simulink model "ILC_CTC"  (R2023b)
settings: Solver=VariableStepAuto  StartTime=0.0  StopTime=20  RelTol=1e-3
values from neighbouring files (symbols this model uses):
  C1 = [1 0 0 0]    [ILCadaptable.m]    (also in parametros3.m = [1 0 0 0 0 0])
  C2 = [0 1 0 0]    [ILCadaptable.m]    (also in parametros3.m = [0 0 1 0 0 0])
  Cv1 = [0 1 0 0 0 0]    [parametros3.m]
  Cv2 = [0 0 0 1 0 0]    [parametros3.m]
  ek1_1 = out.ek1    [ILCadaptable.m]    (also in parametros3.m)
  ek2_1 = out.ek2    [ILCadaptable.m]    (also in parametros3.m)
  L1 = 2    [ILCadaptable.m]    (also in parametros3.m)
  L2 = 2    [ILCadaptable.m]    (also in parametros3.m)
undefined symbols (not defined in the file or in its folder): l1, l2
libraries: simulink x2
settings Model: Creator=LENOVO  LastModifiedBy=LENOVO

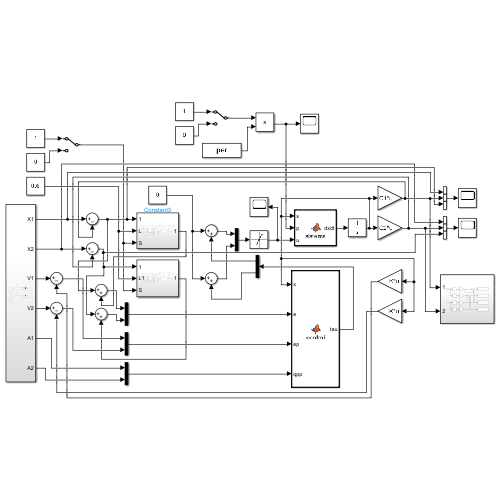
[thumbnail: Simulink's stored preview of the top-level diagram]
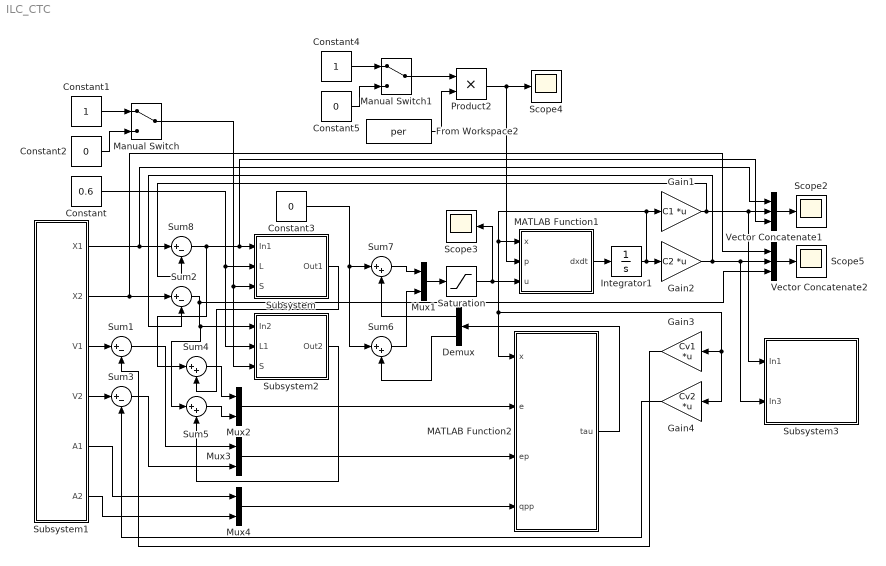
== system ILC_CTC ==
  Constant : Constant  Value=0.6
  Constant1 : Constant
  Constant2 : Constant  Value=0
  Constant3 : Constant  Value=0
  Constant4 : Constant
  Constant5 : Constant  Value=0
  Demux : Demux  Outputs=2
  From Workspace2 : FromWorkspace  VariableName=per
  Gain1 : Gain  Gain=C1  Multiplication=Matrix(K*u)
  Gain2 : Gain  Gain=C2  Multiplication=Matrix(K*u)
  Gain3 : Gain  Gain=Cv1  Multiplication=Matrix(K*u)
  Gain4 : Gain  Gain=Cv2  Multiplication=Matrix(K*u)
  Integrator1 : Integrator  InitialCondition=[0 0 0 0]
  MATLAB Function1 : MATLAB Function  TreatAsAtomicUnit=on
  MATLAB Function2 : MATLAB Function  TreatAsAtomicUnit=on
  Manual Switch : ManualSwitch
  Manual Switch1 : ManualSwitch
  Mux{1..4} (4 alike) : Mux  Inputs=2
  Product2 : Product
  Saturation : Saturate  UpperLimit=2.5  LowerLimit=-2.5
  Scope{2..5} (4 alike) : Scope
  Subsystem : Subsystem
  Subsystem1 : Subsystem
  Subsystem2 : Subsystem
  Subsystem3 : Subsystem
  Sum{1..3,8} (4 alike) : Sum  Inputs=|+-
  Sum{4..7} (4 alike) : Sum  Inputs=|++
  Vector Concatenate1 : Concatenate  NumInputs=3
  Vector Concatenate2 : Concatenate  NumInputs=3
  wires:
  Gain1/1 -> Sum8/2, Subsystem3/1(In1), Vector Concatenate1/2
  Saturation/1 -> Scope3/1, MATLAB Function1/3(u)
  Sum2/1 -> Sum5/1, Subsystem2/1(In2), Vector Concatenate2/3
  Constant1/1 -> Manual Switch/1
  MATLAB Function1/1(dxdt) -> Integrator1/1
  Gain2/1 -> Subsystem3/2(In3), Vector Concatenate2/2, Sum2/2
  Subsystem1/2(X2) -> Sum2/1, Vector Concatenate2/1
  Sum7/1 -> Mux1/1
  Integrator1/1 -> Gain4/1, Gain3/1, MATLAB Function2/1(x), MATLAB Function1/1(x), Gain1/1, Gain2/1
  Vector Concatenate2/1 -> Scope5/1
  Subsystem1/1(X1) -> Vector Concatenate1/1, Sum8/1
  Constant/1 -> Subsystem2/2(L1), Subsystem/2(L)
  Constant2/1 -> Manual Switch/2
  Mux1/1 -> Saturation/1
  Sum8/1 -> Sum4/1, Subsystem/1(In1), Vector Concatenate1/3
  Sum6/1 -> Mux1/2
  Vector Concatenate1/1 -> Scope2/1
  Manual Switch/1 -> Subsystem2/3(S), Subsystem/3(S)
  Subsystem1/3(V1) -> Sum1/1
  Subsystem1/4(V2) -> Sum3/1
  Sum1/1 -> Mux3/1
  Sum3/1 -> Mux3/2
  Subsystem1/5(A1) -> Mux4/1
  Subsystem1/6(A2) -> Mux4/2
  Mux2/1 -> MATLAB Function2/2(e)
  Mux3/1 -> MATLAB Function2/3(ep)
  Mux4/1 -> MATLAB Function2/4(qpp)
  Gain3/1 -> Sum1/2
  Gain4/1 -> Sum3/2
  MATLAB Function2/1(tau) -> Demux/1
  Demux/1 -> Sum7/2
  Demux/2 -> Sum6/2
  Constant3/1 -> Sum6/1, Sum7/1
  Subsystem/1(Out1) -> Sum4/2
  Subsystem2/1(Out2) -> Sum5/2
  Sum4/1 -> Mux2/1
  Sum5/1 -> Mux2/2
  Constant5/1 -> Manual Switch1/2
  Constant4/1 -> Manual Switch1/1
  Manual Switch1/1 -> Product2/1
  From Workspace2/1 -> Product2/2
  Product2/1 -> Scope4/1, MATLAB Function1/2(p)

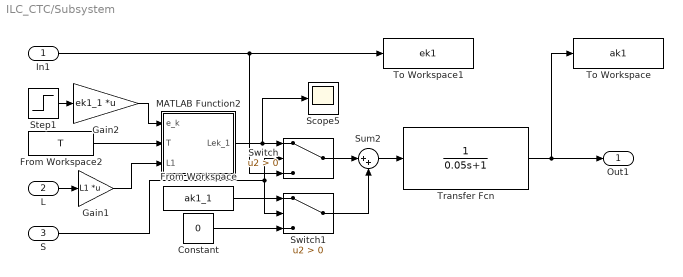
== system ILC_CTC/Subsystem ==
  In1 : Inport
  L : Inport  Port=2
  S : Inport  Port=3
  Constant : Constant  Value=0
  From Workspace : FromWorkspace  VariableName=ak1_1
  From Workspace2 : FromWorkspace  VariableName=T
  Gain1 : Gain  Gain=L1  Multiplication=Matrix(K*u)
  Gain2 : Gain  Gain=ek1_1  Multiplication=Matrix(K*u)
  MATLAB Function2 : MATLAB Function  TreatAsAtomicUnit=on
  Scope5 : Scope
  Step1 : Step  Time=0  SampleTime=0
  Sum2 : Sum  Inputs=|++
  Switch : Switch  Criteria=u2 > Threshold  SaturateOnIntegerOverflow=off  InputSameDT=off
  Switch1 : Switch  Criteria=u2 > Threshold  SaturateOnIntegerOverflow=off  InputSameDT=off
  To Workspace : ToWorkspace  VariableName=ak1  SampleTime=-1
  To Workspace1 : ToWorkspace  VariableName=ek1  SampleTime=-1
  Transfer Fcn : TransferFcn  Denominator=[0.05 1]
  Out1 : Outport
  wires:
  From Workspace2/1 -> MATLAB Function2/2(T)
  In1/1 -> Switch/3, To Workspace1/1
  Gain2/1 -> MATLAB Function2/1(e_k)
  Step1/1 -> Gain2/1
  Constant/1 -> Switch1/3
  MATLAB Function2/1(Lek_1) -> Scope5/1, Switch/1
  Sum2/1 -> Transfer Fcn/1
  Switch1/1 -> Sum2/2
  From Workspace/1 -> Switch1/1
  Switch/1 -> Sum2/1
  Transfer Fcn/1 -> To Workspace/1, Out1/1
  L/1 -> Gain1/1
  S/1 -> Switch1/2, Switch/2
  Gain1/1 -> MATLAB Function2/3(L1)

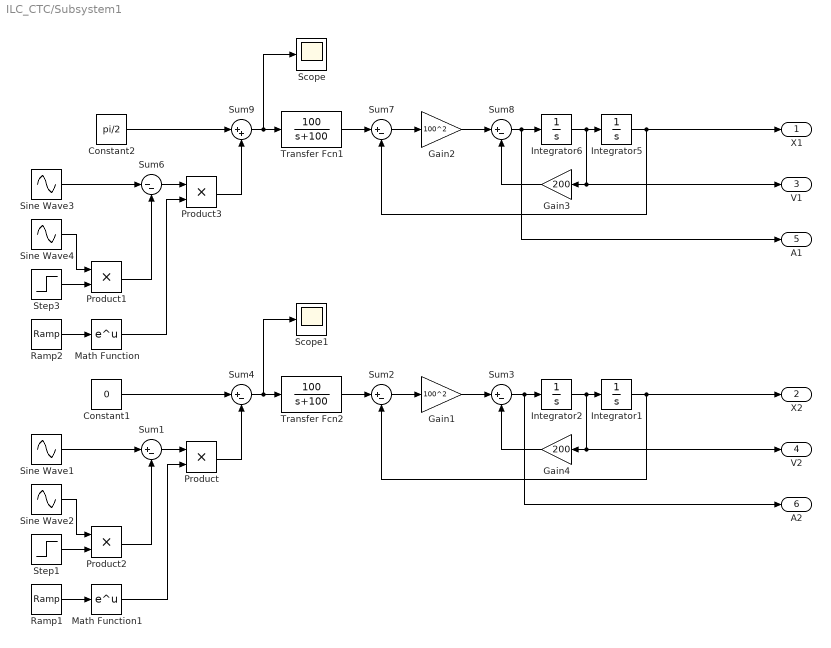
== system ILC_CTC/Subsystem1 ==
  Constant1 : Constant  Value=0
  Constant2 : Constant  Value=pi/2
  Gain1 : Gain  Gain=100^2
  Gain2 : Gain  Gain=100^2
  Gain3 : Gain  Gain=200
  Gain4 : Gain  Gain=200
  Integrator{1..2,5..6} (4 alike) : Integrator
  Math Function : Math
  Math Function1 : Math
  Product{,1..3} (4 alike) : Product
  Ramp1 : simulink/Sources/Ramp  slope=0  start=10  InitialOutput=0
  Ramp2 : simulink/Sources/Ramp  slope=0  start=10  InitialOutput=0
  Scope : Scope
  Scope1 : Scope
  Sine Wave{1..4} (4 alike) : Sin  Frequency=1.5  SampleTime=0
  Step1 : Step  Time=0  After=0  SampleTime=0
  Step3 : Step  Time=0  After=0  SampleTime=0
  Sum{1..4,7..8} (6 alike) : Sum  Inputs=|+-
  Sum6 : Sum  Inputs=|--
  Sum9 : Sum  Inputs=|++
  Transfer Fcn1 : TransferFcn  Numerator=[100]  Denominator=[1 100]
  Transfer Fcn2 : TransferFcn  Numerator=[100]  Denominator=[1 100]
  X1 : Outport
  X2 : Outport  Port=2
  V1 : Outport  Port=3
  V2 : Outport  Port=4
  A1 : Outport  Port=5
  A2 : Outport  Port=6
  wires:
  Sine Wave3/1 -> Sum6/1
  Sum7/1 -> Gain2/1
  Sum8/1 -> A1/1, Integrator6/1
  Sine Wave4/1 -> Product1/1
  Gain2/1 -> Sum8/1
  Transfer Fcn1/1 -> Sum7/1
  Gain3/1 -> Sum8/2
  Product1/1 -> Sum6/2
  Step3/1 -> Product1/2
  Constant2/1 -> Sum9/1
  Integrator6/1 -> Gain3/1, V1/1, Integrator5/1
  Sum9/1 -> Scope/1, Transfer Fcn1/1
  Sum4/1 -> Scope1/1, Transfer Fcn2/1
  Sum3/1 -> A2/1, Integrator2/1
  Gain1/1 -> Sum3/1
  Transfer Fcn2/1 -> Sum2/1
  Sum2/1 -> Gain1/1
  Step1/1 -> Product2/2
  Constant1/1 -> Sum4/1
  Integrator1/1 -> X2/1, Sum2/2
  Sine Wave1/1 -> Sum1/1
  Gain4/1 -> Sum3/2
  Integrator2/1 -> V2/1, Gain4/1, Integrator1/1
  Product2/1 -> Sum1/2
  Sine Wave2/1 -> Product2/1
  Math Function/1 -> Product3/2
  Math Function1/1 -> Product/2
  Ramp2/1 -> Math Function/1
  Ramp1/1 -> Math Function1/1
  Sum6/1 -> Product3/1
  Product3/1 -> Sum9/2
  Sum1/1 -> Product/1
  Product/1 -> Sum4/2
  Integrator5/1 -> Sum7/2, X1/1

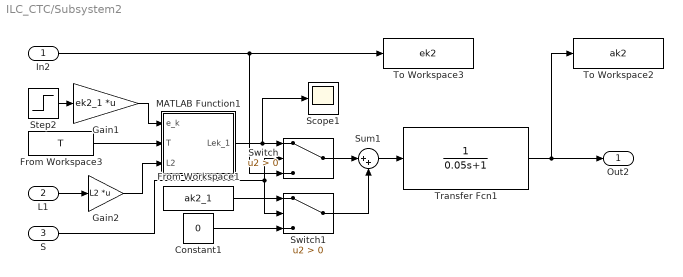
== system ILC_CTC/Subsystem2 ==
  In2 : Inport
  L1 : Inport  Port=2
  S : Inport  Port=3
  Constant1 : Constant  Value=0
  From Workspace1 : FromWorkspace  VariableName=ak2_1
  From Workspace3 : FromWorkspace  VariableName=T
  Gain1 : Gain  Gain=ek2_1  Multiplication=Matrix(K*u)
  Gain2 : Gain  Gain=L2  Multiplication=Matrix(K*u)
  MATLAB Function1 : MATLAB Function  TreatAsAtomicUnit=on
  Scope1 : Scope
  Step2 : Step  Time=0  SampleTime=0
  Sum1 : Sum  Inputs=|++
  Switch : Switch  Criteria=u2 > Threshold  SaturateOnIntegerOverflow=off  InputSameDT=off
  Switch1 : Switch  Criteria=u2 > Threshold  SaturateOnIntegerOverflow=off  InputSameDT=off
  To Workspace2 : ToWorkspace  VariableName=ak2  SampleTime=-1
  To Workspace3 : ToWorkspace  VariableName=ek2  SampleTime=-1
  Transfer Fcn1 : TransferFcn  Denominator=[0.05 1]
  Out2 : Outport
  wires:
  MATLAB Function1/1(Lek_1) -> Scope1/1, Switch/1
  S/1 -> Switch1/2, Switch/2
  Sum1/1 -> Transfer Fcn1/1
  Gain1/1 -> MATLAB Function1/1(e_k)
  Transfer Fcn1/1 -> To Workspace2/1, Out2/1
  In2/1 -> Switch/3, To Workspace3/1
  From Workspace1/1 -> Switch1/1
  From Workspace3/1 -> MATLAB Function1/2(T)
  Constant1/1 -> Switch1/3
  Step2/1 -> Gain1/1
  Switch1/1 -> Sum1/2
  Switch/1 -> Sum1/1
  L1/1 -> Gain2/1
  Gain2/1 -> MATLAB Function1/3(L2)

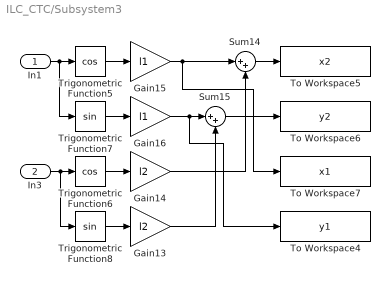
== system ILC_CTC/Subsystem3 ==
  In1 : Inport
  In3 : Inport  Port=2
  Gain13 : Gain  Gain=l2
  Gain14 : Gain  Gain=l2
  Gain15 : Gain  Gain=l1
  Gain16 : Gain  Gain=l1
  Sum14 : Sum  Inputs=|++
  Sum15 : Sum  Inputs=|++
  To Workspace4 : ToWorkspace  VariableName=y1  SaveFormat=Timeseries  SampleTime=-1
  To Workspace5 : ToWorkspace  VariableName=x2  SaveFormat=Timeseries  SampleTime=-1
  To Workspace6 : ToWorkspace  VariableName=y2  SaveFormat=Timeseries  SampleTime=-1
  To Workspace7 : ToWorkspace  VariableName=x1  SaveFormat=Timeseries  SampleTime=-1
  Trigonometric Function5 : Trigonometry  Operator=cos
  Trigonometric Function6 : Trigonometry  Operator=cos
  Trigonometric Function7 : Trigonometry
  Trigonometric Function8 : Trigonometry
  wires:
  Trigonometric Function6/1 -> Gain14/1
  Sum15/1 -> To Workspace6/1
  Trigonometric Function8/1 -> Gain13/1
  Gain13/1 -> Sum15/2
  Sum14/1 -> To Workspace5/1
  Gain14/1 -> Sum14/2
  Trigonometric Function5/1 -> Gain15/1
  Gain16/1 -> To Workspace4/1, Sum15/1
  Gain15/1 -> Sum14/1, To Workspace7/1
  Trigonometric Function7/1 -> Gain16/1
  In3/1 -> Trigonometric Function8/1, Trigonometric Function6/1
  In1/1 -> Trigonometric Function7/1, Trigonometric Function5/1

== matlab function ILC_CTC/MATLAB Function1 ==
  data: x input; p input; u input; dxdt output
function dxdt = sistema(x,p,u)

%definición de parametros
m1 = 0.066;
m2 = 0.0792;
lc1 = 0.125;
lc2 = 0.15;
l1 = 0.25;
l2 = 0.3;
I1 = 0.00138;
I2 = 0.00238;
g = 9.81;

%calculo de las constantes del sistema
a1 = m1*lc1^2+m2*l1^2+I1;
a2 = m2*lc2^2+I2;
a3 = m2*l1*lc2;
a4 = m1*lc1+m2*l1;
a5 = m2*lc2;

%Perturbación paramétrica
a1=a1+p(1)
a2=a2+p(2)
a3=a3+p(3)
a4=a4+p(4)
a5=a5+p(5)

%variables de estado
x1 = x(1);
x2 = x(2);
x3 = x(3);
x4 = x(4);

%Matrices del sistema
G = [a4*g*cos(x1)+a5*g*cos(x1+x3);a5*g*cos(x1+x3)];%matriz de gravedad 
C = [-2*a3*sin(x3)*x4 -a3*sin(x3)*x4;
     a3*sin(x3)*x2 0];%matriz de velocidad o coriolis
M = [a1+a2+2*a3*cos(x3) a2+a3*cos(x3);
     a2+a3*cos(x3) a2];%matriz de aceleración

%d/dt[x1;x2;x3;x4]=[f1;f2;f3;f4]
%calculo de f2 y f4 
xb = M^(-1)*u-M^(-1)*C*[x2;x4]-M^(-1)*G;

%sistema en la forma d/dt[x1;x2;x3;x4]=[f1;f2;f3;f4] 
dxdt = [x2; 
        xb(1);
        x4;
        xb(2)];

== matlab function ILC_CTC/Subsystem/MATLAB Function2 ==
  data: Lek_1 output; e_k input; T input; L1 input
function Lek_1 = noncausal(e_k,T,L1)
n = int32(T);
Lek_1 = L1*(e_k(n+1) - e_k(n))/0.03;

== matlab function ILC_CTC/MATLAB Function2 ==
  data: x input; e input; ep input; qpp input; tau output
function tau = control(x,e,ep,qpp)

%constantes del controlador
kp = 15;
kv = 10;

%definición de parametros
m1 = 0.066;
m2 = 0.0792;
lc1 = 0.125;
lc2 = 0.15;
l1 = 0.25;
l2 = 0.3;
I1 = 0.00138;
I2 = 0.00238;
g = 9.81;

%calculo de las constantes del sistema
a1 = m1*lc1^2+m2*l1^2+I1;
a2 = m2*lc2^2+I2;
a3 = m2*l1*lc2;
a4 = m1*lc1+m2*l1;
a5 = m2*lc2;

%variables de estado
x1 = x(1);
x2 = x(2);
x3 = x(3);
x4 = x(4);

%Matrices del sistema
G = [a4*g*cos(x1)+a5*g*cos(x1+x3);a5*g*cos(x1+x3)];%matriz de gravedad 
C = [-2*a3*sin(x3)*x4 -a3*sin(x3)*x4;
     a3*sin(x3)*x2 0];%matriz de velocidad o coriolis
M = [a1+a2+2*a3*cos(x3) a2+a3*cos(x3);
     a2+a3*cos(x3) a2];%matriz de aceleración

%calculo de accion de control
tau = M*(qpp+kp*e+kv*ep)+C*[x2;x4]+G;

== matlab function ILC_CTC/Subsystem2/MATLAB Function1 ==
  data: Lek_1 output; e_k input; T input; L2 input
function Lek_1 = noncausal(e_k,T,L2)
n = int32(T);
Lek_1 = L2*(e_k(n+1) - e_k(n))/0.03;
